simulink model "QD2_MissionCtrl_Hover_2021a"  (R2026a)
settings: Solver=ode2  StopTime=inf  FixedStep=0.001  EnableMultiTasking=on
undefined symbols (not defined in the file): _MissionCtrl, datetime, Host, log_, m, qc_get_step_size, saved_data
libraries: quarc_library x29, simulink x10, simulink_extras x1
(part 2 of 2)

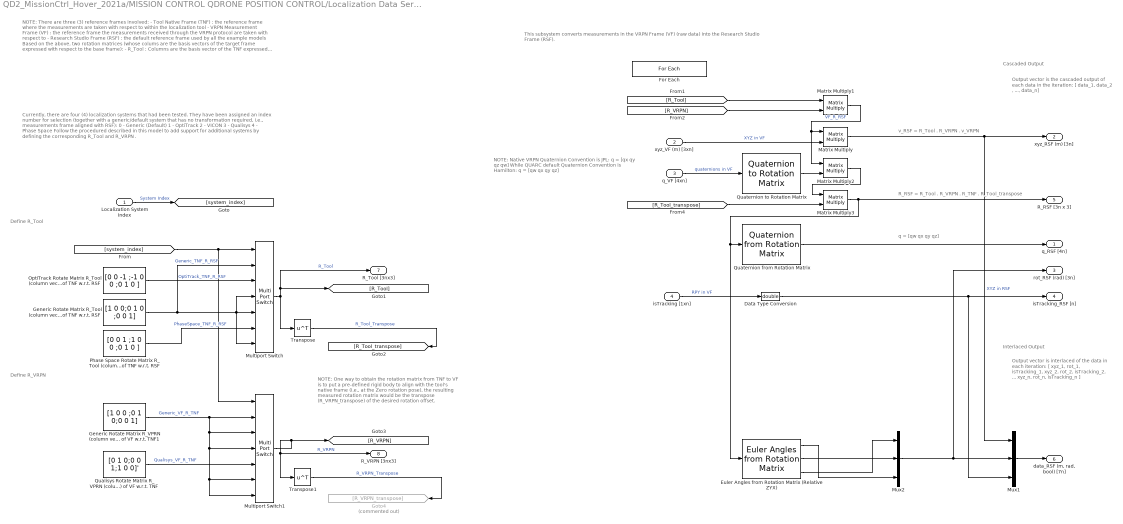
== system QD2_MissionCtrl_Hover_2021a/MISSION CONTROL QDRONE POSITION CONTROL/Localization Data Server (VRPN) /For Each Subsystem (Convention Correction: Motive Frame to Research Studio Frame)1 ==
  note: This subsystem converts measurements in the VRPN Frame (VF) (raw data) into the Research Studio Frame (RSF).
  note: q = [qw qx qy qz]
  note: Cascaded Output
  note: Output vector is the cascaded output of
      | each data in the iteration:
      | [ data_1, data_2 , ..., data_n]
  note: Interlaced Output
  note: Output vector is interlaced of the data
      | in each iteration:
      |
      | [ xyz_1, rot_1, isTracking_1,
      |   xyz_2, rot_2, isTracking_2,
      |   ...
      |   xyz_n, rot_n, isTracking_n ]
  note: NOTE: Native VRPN Quaternion Convention is JPL:
      | q = [qx qy qz qw]
      |
      | While QUARC default Quaternion Convention is Hamilton:
      | q = [qw qx qy qz]
  note: NOTE:
      | One way to obtain the rotation matrix from TNF to VF
      | is to put a pre-defined rigid body to align with the tool's
      | native frame (i.e., at the Zero rotation pose), the resulting
      | measured rotation matrix would be the transpose (R_VRPN_transpose) of the desired rotation
      | offset.
  note: NOTE:
      | There are three (3) reference frames involved:
      |
      | - Tool Native Frame (TNF) : the reference frame where the measurements are taken with respect to within the localization tool
      | - VRPN Measurement Frame (VF) : the reference frame the measurements received through the VRPN protocol are taken with respect to
      | - Research Studio Frame (RSF) : the default reference frame used by all the example models
      |
      | Based on the above, two rotation matrices (whose colums are the basis vectors of the target frame expressed with respect to the base frame):
      |
      | - R_Tool : Columns are the basis vector of the TNF expressed with respect to the RSF
      | - R_VPRN : Columns are the basis vector of the VRPN frame with respect to the TNF
      |
      | If all of the reference are aligned, then both R_Tool and R_VRPN will be a 3x3 identity matrices.
  note: Define R_Tool
  note: Currently, there are four (4) localization systems that had been tested. They have been assigned an index number for selection (together with a generic/default system that has no transformation required, i.e., measurements frame aligned with RSF):
      |
      | 0 - Generic (Default)
      | 1 - OptiTrack
      | 2 - VICON
      | 3 - Qualisys
      | 4 - Phase Space
      |
      | Follow the procedured described in this model to add support for additional systems by defining the corresponding R_Tool and R_VRPN .
  note: Define R_VRPN
  note: v_RSF = R_Tool . R_VRPN . v_VRPN
  note: R_RSF = R_Tool . R_VRPN . R_TNF . R_Tool_transpose
  Localization System Index : Inport
  xyz_VF (m) [3xn] : Inport  Port=2  Partition=on  PartitionDimension=2  PartitionWidth=1  PartitionOffset=0
  q_VF [4xn] : Inport  Port=3  Partition=on  PartitionDimension=2  PartitionWidth=1  PartitionOffset=0
  isTracking [1xn] : Inport  Port=4  Partition=on  PartitionDimension=2  PartitionWidth=1  PartitionOffset=0
  " Generic Rotate Matrix R_VPRN (column vectors are basis vectors) of VF w.r.t. TNF1" : Constant  Value=[1 0 0 ;0 1 0;0 0 1]  VectorParams1D=off
  " Qualisys Rotate Matrix R_VPRN (column vectors are basis vectors) of VF w.r.t. TNF" : Constant  Value=[0 1 0;0 0 1;1 0 0]'  VectorParams1D=off
  Data Type Conversion : DataTypeConversion  OutDataTypeStr=double  SaturateOnIntegerOverflow=off  RndMeth=Floor
  Euler Angles from Rotation Matrix (Relative ZYX) : quarc_library/Math Operations/Matrices/Euler Angles from Rotation Matrix  menu_order=Relative Z-Y-X
      settings: SourceProductName=QUARC Targets
  For Each : ForEach  DisableCoverage=on
  Generic Rotate Matrix R_Tool (column vectors are basis vectors) of TNF w.r.t. RSF : Constant  Value=[1 0 0;0 1 0 ;0 0 1]  VectorParams1D=off
  Goto4 : Goto  Commented=on  GotoTag=R_VRPN_transpose
  Matrix Multiply{,1..3} (4 alike) : Product  Multiplication=Matrix(*)
  Multiport Switch : MultiPortSwitch  DataPortOrder=Zero-based contiguous  Inputs=5  DataPortForDefault=Additional data port  DiagnosticForDefault=None  zeroidx=on  SaturateOnIntegerOverflow=off  InputSameDT=off
  Multiport Switch1 : MultiPortSwitch  DataPortOrder=Zero-based contiguous  Inputs=5  DataPortForDefault=Additional data port  DiagnosticForDefault=None  zeroidx=on  SaturateOnIntegerOverflow=off  InputSameDT=off
  Mux1 : Mux  Inputs=3
  Mux2 : Mux  Inputs=3
  OptiTrack Rotate Matrix R_Tool (column vectors are basis vectors) of TNF w.r.t. RSF : Constant  Value=[0 0 -1 ;-1 0 0 ;0 1 0 ]  VectorParams1D=off
  Phase Space Rotate Matrix R_Tool (column vectors are basis vectors) of TNF w.r.t. RSF : Constant  Value=[0 0 1 ;1 0 0 ;0 1 0 ]  VectorParams1D=off
  Quaternion from Rotation Matrix : quarc_library/Math Operations/Quaternions/Quaternion from Rotation Matrix
      settings: SourceProductName=QUARC Targets
  Quaternion to Rotation Matrix : quarc_library/Math Operations/Quaternions/Quaternion to Rotation Matrix
      settings: SourceProductName=QUARC Targets
  Transpose : Math  Operator=transpose
  Transpose1 : Math  Operator=transpose
  q_RSF [4n] : Outport  ConcatenationDimension=1
  xyz_RSF (m) [3n] : Outport  Port=2  ConcatenationDimension=1
  rot_RSF (rad) [3n] : Outport  Port=3  ConcatenationDimension=1
  isTracking_RSF [n] : Outport  Port=4  ConcatenationDimension=1
  R_RSF [3n x 3] : Outport  Port=5  ConcatenationDimension=1
  "data_RSF (m, rad, bool) [7n]" : Outport  Port=6  ConcatenationDimension=1
  R_Tool [3nx3] : Outport  Port=7  ConcatenationDimension=1
  R_VRPN [3nx3] : Outport  Port=8  ConcatenationDimension=1
  wires:
  Phase Space Rotate Matrix R_Tool (column vectors are basis vectors) of TNF w.r.t. RSF/1 -> Multiport Switch/6  "PhaseSpace_TNF_R_RSF"
  Localization System Index/1 -> [system_index]  "System Index"
  Matrix Multiply3/1 -> R_RSF [3n x 3]/1, Quaternion from Rotation Matrix/1, Euler Angles from Rotation Matrix (Relative ZYX)/1
  [R_Tool_transpose] -> Matrix Multiply3/2
  Matrix Multiply1/1 -> Matrix Multiply/1, Matrix Multiply2/1  "VF_R_RSF"
  [R_VRPN] -> Matrix Multiply1/2
  [R_Tool] -> Matrix Multiply1/1
  Transpose1/1 -> Goto4/1  "R_VRPN_Transpose"
  Multiport Switch1/1 -> [R_VRPN], Transpose1/1, R_VRPN [3nx3]/1  "R_VRPN"
  Transpose/1 -> [R_Tool_transpose]  "R_Tool_Transpose"
  Multiport Switch/1 -> Transpose/1, [R_Tool], R_Tool [3nx3]/1  "R_Tool"
  [system_index] -> Multiport Switch/1, Multiport Switch1/1
  " Qualisys Rotate Matrix R_VPRN (column vectors are basis vectors) of VF w.r.t. TNF"/1 -> Multiport Switch1/5  "Qualisys_VF_R_TNF"
  " Generic Rotate Matrix R_VPRN (column vectors are basis vectors) of VF w.r.t. TNF1"/1 -> Multiport Switch1/2, Multiport Switch1/3, Multiport Switch1/4, Multiport Switch1/7, Multiport Switch1/6  "Generic_VF_R_TNF"
  OptiTrack Rotate Matrix R_Tool (column vectors are basis vectors) of TNF w.r.t. RSF/1 -> Multiport Switch/3  "OptiTrack_TNF_R_RSF"
  Generic Rotate Matrix R_Tool (column vectors are basis vectors) of TNF w.r.t. RSF/1 -> Multiport Switch/2, Multiport Switch/7, Multiport Switch/5, Multiport Switch/4  "Generic_TNF_R_RSF"
  Quaternion from Rotation Matrix/1 -> q_RSF [4n]/1
  Matrix Multiply2/1 -> Matrix Multiply3/1
  Quaternion to Rotation Matrix/1 -> Matrix Multiply2/2
  Mux2/1 -> rot_RSF (rad) [3n]/1, Mux1/2
  Euler Angles from Rotation Matrix (Relative ZYX)/2 -> Mux2/2
  Euler Angles from Rotation Matrix (Relative ZYX)/1 -> Mux2/3
  Euler Angles from Rotation Matrix (Relative ZYX)/3 -> Mux2/1
  Data Type Conversion/1 -> isTracking_RSF [n]/1, Mux1/3
  Mux1/1 -> "data_RSF (m, rad, bool) [7n]"/1
  isTracking [1xn]/1 -> Data Type Conversion/1  "RPY in VF"
  xyz_VF (m) [3xn]/1 -> Matrix Multiply/2  "XYZ in VF"
  Matrix Multiply/1 -> Mux1/1, xyz_RSF (m) [3n]/1  "XYZ in RSF"
  q_VF [4xn]/1 -> Quaternion to Rotation Matrix/1  "quaternions in VF"

== system QD2_MissionCtrl_Hover_2021a/MISSION CONTROL QDRONE POSITION CONTROL/JOYSTICK_FRSKY/Pulse Check/pulse count  ==
  Trigger : TriggerPort  VariantControl=Variant
  Constant1 : Constant  Value=0
  Increment Stored Integer : simulink/Additional Math & Discrete/Additional Math: Increment - Decrement/Increment Stored Integer
  Sum : Sum  Inputs=|++
  Unit Delay : UnitDelay  SampleTime=-1
  Number of Pulses : Outport  VectorParamsAs1DForOutWhenUnconnected=off
  wires:
  Constant1/1 -> Sum/1
  Sum/1 -> Increment Stored Integer/1
  Unit Delay/1 -> Sum/2
  Increment Stored Integer/1 -> Unit Delay/1, Number of Pulses/1

== system QD2_MissionCtrl_Hover_2021a/MISSION CONTROL QDRONE POSITION CONTROL/JOYSTICK_SPEKTRUM/Pulse Check/pulse count  ==
  Trigger : TriggerPort  VariantControl=Variant
  Constant1 : Constant  Value=0
  Increment Stored Integer : simulink/Additional Math & Discrete/Additional Math: Increment - Decrement/Increment Stored Integer
  Sum : Sum  Inputs=|++
  Unit Delay : UnitDelay  SampleTime=-1
  Number of Pulses : Outport  VectorParamsAs1DForOutWhenUnconnected=off
  wires:
  Constant1/1 -> Sum/1
  Sum/1 -> Increment Stored Integer/1
  Unit Delay/1 -> Sum/2
  Increment Stored Integer/1 -> Unit Delay/1, Number of Pulses/1

== matlab function QD2_MissionCtrl_Hover_2021a/MISSION CONTROL QDRONE POSITION CONTROL/Subsystem/MATLAB Function ==
  data: Arm input; Flight_State output; Takeoff_Land_Flag input; Emergency_Stop input; Joystick_Issue input; Stop_MS output; Communication_Issue input
function [Flight_State, Stop_MS]= Flight_Plan(Arm, ...
                            Takeoff_Land_Flag, ...
                            Emergency_Stop, ...
                            Joystick_Issue, ...
                            Communication_Issue)

persistent State

if isempty(State);
    State = 0;

end 
Stop_MS = 0;


switch State 

    case 0 % ============== QDrone Idle Sate ============== 
            
        if  Arm == 1 & Emergency_Stop == 0 && Joystick_Issue == 0
            State = 1;
        elseif Joystick_Issue == 1 || Emergency_Stop == 1 || Takeoff_Land_Flag == 1 || Communication_Issue == 1
            State = 9 ;
        end 

    case 1 % ============== QDrone Armed Sate ============== 
          if Emergency_Stop == 0 && Joystick_Issue == 0 
               if Arm == 0 
                     State = 0 ;
               elseif Arm == 1 && Takeoff_Land_Flag == 1 
                     State = 2 ;
                 end
              elseif Joystick_Issue == 1 || Communication_Issue == 1 || Emergency_Stop == 1
                State = 9 ;
        end 
          
    case 2 % ============== QDrone Takeoff Sate ============== 
          if Emergency_Stop == 0 && Joystick_Issue == 0 
               if Takeoff_Land_Flag == 0 
                State = 3 ;
              elseif Joystick_Issue == 1 || Arm == 0 || Communication_Issue == 1|| Emergency_Stop == 1
                State = 9 ;
               end 
          end 

    case 3 % ============== QDrone Land Sate ============== 
           if Joystick_Issue == 1 || Arm == 0 || Communication_Issue == 1
               State = 9 ;
           end

    case 9 % ============== MS Stop Sate ============== 
            Stop_MS = 1;
    
end 

Flight_State = State ;

== matlab function QD2_MissionCtrl_Hover_2021a/Communication/Detect Communication loss/MATLAB Function ==
  data: time input; stream_connection_loss output; state input; error input
function stream_connection_loss  = fcn(time, state, error)

stream_connection_loss = 0;
if time > 1
    if ~((state == 2)&&(error >= 0))
        % stream connection is not established correctly
        stream_connection_loss = 1;
    end
end
